simulink model "FilterEX_3"  (R2020b)
settings: Solver=FixedStepAuto  StartTime=0.0  StopTime=0.05  FixedStep=0.000002  RelTol=1e-3
values from neighbouring files (symbols this model uses):
  d = 10109.66    [DATA.mat]
  k = 10000    [DATA.mat]
  r = 9890.34    [DATA.mat]
settings Model: Creator=JAGRUTI SHINDE  LastModifiedBy=JAGRUTI SHINDE

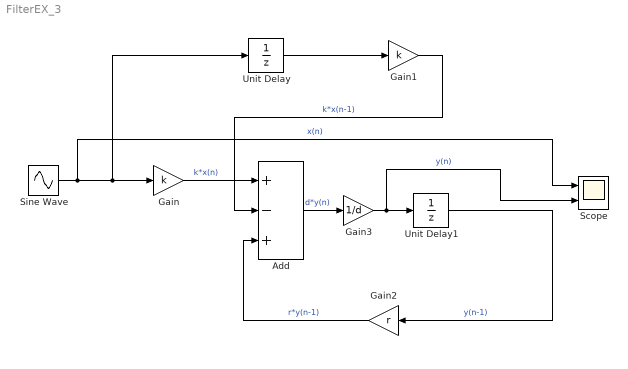
== system FilterEX_3 ==
  Add : Sum  Inputs=+-+
  Gain : Gain  Gain=k
  Gain1 : Gain  Gain=k
  Gain2 : Gain  Gain=r
  Gain3 : Gain  Gain=1/d
  Scope : Scope  NumInputPorts=2
  Sine Wave : Sin  Frequency=2*pi*500  SampleTime=0
  Unit Delay : UnitDelay  SampleTime=-1  HasFrameUpgradeWarning=on
  Unit Delay1 : UnitDelay  SampleTime=-1  HasFrameUpgradeWarning=on
  wires:
  Gain/1 -> Add/1  "k*x(n)"
  Sine Wave/1 -> Scope/1, Unit Delay/1, Gain/1  "x(n)"
  Unit Delay/1 -> Gain1/1
  Gain1/1 -> Add/2  "k*x(n-1)"
  Unit Delay1/1 -> Gain2/1  "y(n-1)"
  Gain2/1 -> Add/3  "r*y(n-1)"
  Gain3/1 -> Scope/2, Unit Delay1/1  "y(n)"
  Add/1 -> Gain3/1  "d*y(n)"
